simulink model "recursive"  (R2023b)
settings: Solver=VariableStepAuto  StartTime=0.0  StopTime=10.0  RelTol=1e-3
undefined symbols (not defined in the file): a1, a2, a3, b0, b1, b2, b3
settings Model: Creator=eechris  LastModifiedBy=eechris

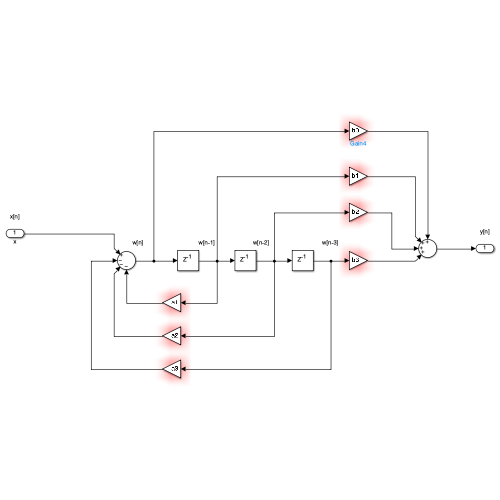
[thumbnail: Simulink's stored preview of the top-level diagram]
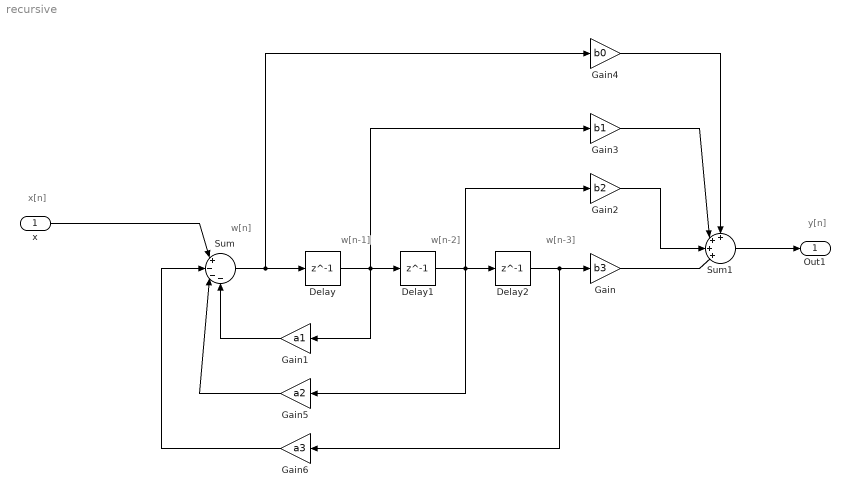
== system recursive ==
  note: w[n]
  note: x[n]
  note: y[n]
  note: w[n-1]
  note: w[n-2]
  note: w[n-3]
  x : Inport
  Delay : Delay  DelayLength=1  InitialCondition=0
  Delay1 : Delay  DelayLength=1  InitialCondition=0
  Delay2 : Delay  DelayLength=1  InitialCondition=0
  Gain : Gain  Gain=b3
  Gain1 : Gain  Gain=a1
  Gain2 : Gain  Gain=b2
  Gain3 : Gain  Gain=b1
  Gain4 : Gain  Gain=b0
  Gain5 : Gain  Gain=a2
  Gain6 : Gain  Gain=a3
  Sum : Sum  Inputs=|+---
  Sum1 : Sum  Inputs=++++|
  Out1 : Outport
  wires:
  Delay/1 -> Gain1/1, Gain3/1, Delay1/1
  Delay1/1 -> Gain5/1, Gain2/1, Delay2/1
  Sum/1 -> Delay/1, Gain4/1
  x/1 -> Sum/1
  Delay2/1 -> Gain6/1, Gain/1
  Gain/1 -> Sum1/4
  Gain4/1 -> Sum1/1
  Gain3/1 -> Sum1/2
  Gain2/1 -> Sum1/3
  Gain1/1 -> Sum/4
  Gain5/1 -> Sum/3
  Gain6/1 -> Sum/2
  Sum1/1 -> Out1/1
